simulink model "three_phase_inverter(multi)"  (R2021b)
settings: Solver=FixedStepDiscrete  StartTime=0.0  StopTime=5  FixedStep=1e-6  RelTol=1e-3
libraries: spsIGBTDiodeLib x6, simulink x4, spsVoltageMeasurementLib x4, spsSeriesRLCBranchLib x3, spsCurrentMeasurementLib x1, spsDCVoltageSourceLib x1, spspowerguiLib x1
settings Model: Creator=banof  LastModifiedBy=Devanand Kumar
settings DebuggingCC: UnconnectedInputMsg=none  UnconnectedOutputMsg=none  UnconnectedLineMsg=none
settings ModelReferenceCC: EnableRefExpFcnMdlSchedulingChecks=off
settings RTWCC: DLArmComputeVersion=20.02.1

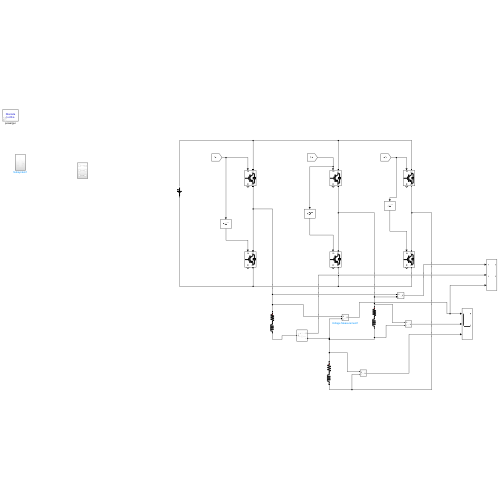
[thumbnail: Simulink's stored preview of the top-level diagram]
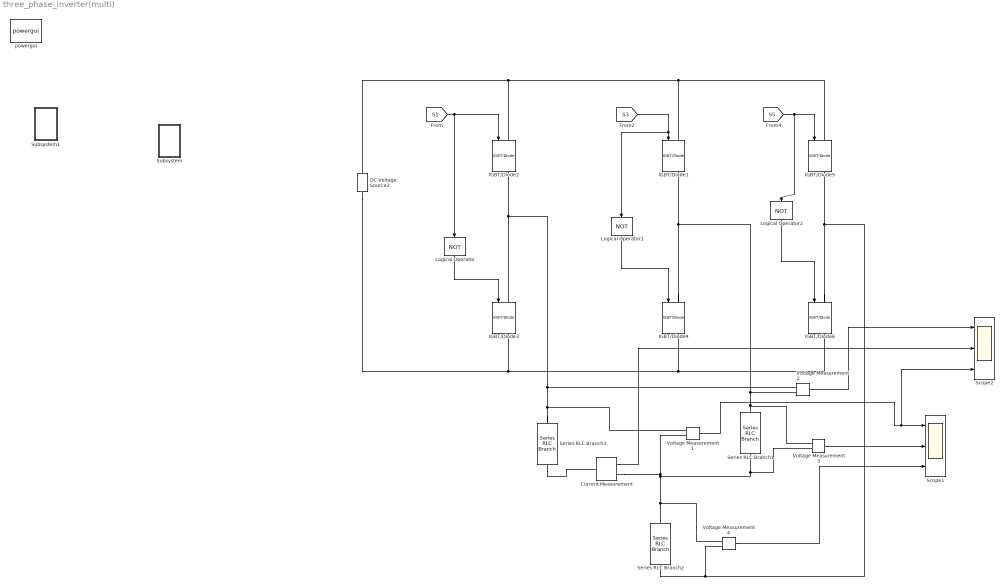
== system three_phase_inverter(multi) ==
  Current Measurement : spsCurrentMeasurementLib/Current Measurement  PhasorSimulation=off  OutputType=Complex  PSBequivalent=0
  DC Voltage Source2 : spsDCVoltageSourceLib/DC Voltage Source  Amplitude=100  Measurements=None
  IGBT/Diode{1..6} (6 alike) : spsIGBTDiodeLib/IGBT//Diode  Ron=1e-3  Rs=1e5  Cs=inf  Measurements=on
  Logical Operator : Logic  Operator=NOT  AllPortsSameDT=off  OutDataTypeStr=boolean
  Logical Operator1 : Logic  Operator=NOT  AllPortsSameDT=off  OutDataTypeStr=boolean
  Logical Operator2 : Logic  Operator=NOT  AllPortsSameDT=off  OutDataTypeStr=boolean
  Scope1 : Scope  NumInputPorts=3
  Scope2 : Scope  NumInputPorts=3
  Series RLC Branch1 : spsSeriesRLCBranchLib/Series RLC Branch  LConnTagsString=__new0  RConnTagsString=__new0  BranchType=RL  Resistance=100  Inductance=100e-3  SetiL0=off  InitialCurrent=0  Capacitance=1e-6  Setx0=off  InitialVoltage=0  Measurements=None
  Series RLC Branch2 : spsSeriesRLCBranchLib/Series RLC Branch  LConnTagsString=__new0  RConnTagsString=__new0  BranchType=RL  Resistance=100  Inductance=100e-3  SetiL0=off  InitialCurrent=0  Capacitance=1e-6  Setx0=off  InitialVoltage=0  Measurements=None
  Series RLC Branch3 : spsSeriesRLCBranchLib/Series RLC Branch  LConnTagsString=__new0  RConnTagsString=__new0  BranchType=RL  Resistance=100  Inductance=100e-3  SetiL0=off  InitialCurrent=0  Capacitance=1e-6  Setx0=off  InitialVoltage=0  Measurements=None
  Subsystem : Subsystem
  Subsystem1 : Subsystem
  Voltage Measurement{1..4} (4 alike) : spsVoltageMeasurementLib/Voltage Measurement  PhasorSimulation=off  OutputType=Complex  PSBequivalent=0
  powergui : spspowerguiLib/powergui  Priority=1  SimulationMode=Discrete  SampleTime=1e-6  frequency=60  Iterations=50  frequencyindice=0  Pbase=100e6  ErrMax=1e-4  UnitsV=kV  UnitsW=MW  buscounter=0  FunctionMessages=off  echomessages=off  EnableUseOfTLC=off  CurrentSourceSwitches=off  DisableSnubberDevices=off  DisableRonSwitches=off  DisableVfSwitches=off  DisplayEquations=off  AutomaticDiscreteSolvers=off  SolverType=Tustin/Backward Euler (TBE)  Interpol=off  ExternalGateDelay=off  methode=off  Ts=100  x0status=blocks  SPID=on  SwTol=0  HookPort=off  NonlinearTolerance=1e-4  nMaxIteration=100  ContinueOnMaxIteration=off  RestoreLinks=warning  ResistiveCurrentMeasurement=off  Frange=[0:2:500]  Ylog=off  Xlog=on  ShowGrid=off  save=off  variable=ZData  structure=0  ZoomFFT=off  StartTime=0.0  cycles=1  DisplayStyle=1  fundamental=60  FreqAxis=off  MaxFrequency=1000  frequencyindicesteady=1  RmsSteady=1  display=off
  wires:
  [S1] -> Logical Operator/1, IGBT/Diode2/1
  Logical Operator/1 -> IGBT/Diode3/1
  [S3] -> Logical Operator1/1, IGBT/Diode1/1
  Logical Operator1/1 -> IGBT/Diode4/1
  Logical Operator2/1 -> IGBT/Diode6/1
  [S5] -> Logical Operator2/1, IGBT/Diode5/1
  Voltage Measurement3/1 -> Scope1/2
  Voltage Measurement1/1 -> Scope2/3, Scope1/1
  Voltage Measurement4/1 -> Scope1/3
  Voltage Measurement2/1 -> Scope2/1
  Current Measurement/1 -> Scope2/2
  connections:
  IGBT/Diode3/RConn1 -- IGBT/Diode6/RConn1 -- IGBT/Diode4/RConn1 -- DC Voltage Source2/LConn1
  IGBT/Diode2/RConn1 -- Voltage Measurement2/LConn1 -- Series RLC Branch3/LConn1 -- Voltage Measurement1/LConn1 -- IGBT/Diode3/LConn1
  DC Voltage Source2/RConn1 -- IGBT/Diode5/LConn1 -- IGBT/Diode1/LConn1 -- IGBT/Diode2/LConn1
  IGBT/Diode4/LConn1 -- Voltage Measurement3/LConn1 -- Series RLC Branch1/LConn1 -- Voltage Measurement2/LConn2 -- IGBT/Diode1/RConn1
  IGBT/Diode6/LConn1 -- Voltage Measurement4/LConn2 -- Series RLC Branch2/RConn1 -- IGBT/Diode5/RConn1
  Voltage Measurement4/LConn1 -- Series RLC Branch2/LConn1 -- Current Measurement/RConn1 -- Voltage Measurement1/LConn2 -- Voltage Measurement3/LConn2 -- Series RLC Branch1/RConn1
  Series RLC Branch3/RConn1 -- Current Measurement/LConn1

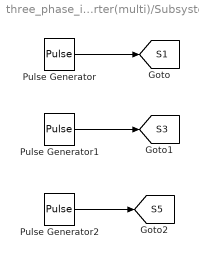
== system three_phase_inverter(multi)/Subsystem ==
  Pulse Generator : DiscretePulseGenerator  Period=20000  PulseWidth=10000  SampleTime=1e-6
  Pulse Generator1 : DiscretePulseGenerator  Period=20000  PulseWidth=10000  PhaseDelay=6666  SampleTime=1e-6
  Pulse Generator2 : DiscretePulseGenerator  Period=20000  PulseWidth=10000  PhaseDelay=13333  SampleTime=1e-6
  tag scope: S1=global, S3=global, S5=global
  wires:
  Pulse Generator/1 -> [S1]
  Pulse Generator2/1 -> [S5]
  Pulse Generator1/1 -> [S3]

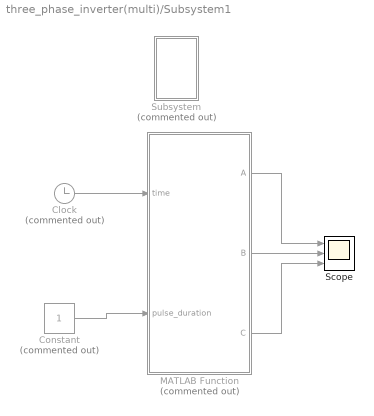
== system three_phase_inverter(multi)/Subsystem1 ==
  Clock : Clock  Commented=on
  Constant : Constant  Commented=on
  MATLAB Function : MATLAB Function  Commented=on  TreatAsAtomicUnit=on
  Scope : Scope  NumInputPorts=3
  Subsystem : Subsystem  Commented=on
  wires:
  MATLAB Function/3(C) -> Scope/3
  Constant/1 -> MATLAB Function/2(pulse_duration)
  MATLAB Function/2(B) -> Scope/2
  MATLAB Function/1(A) -> Scope/1
  Clock/1 -> MATLAB Function/1(time)

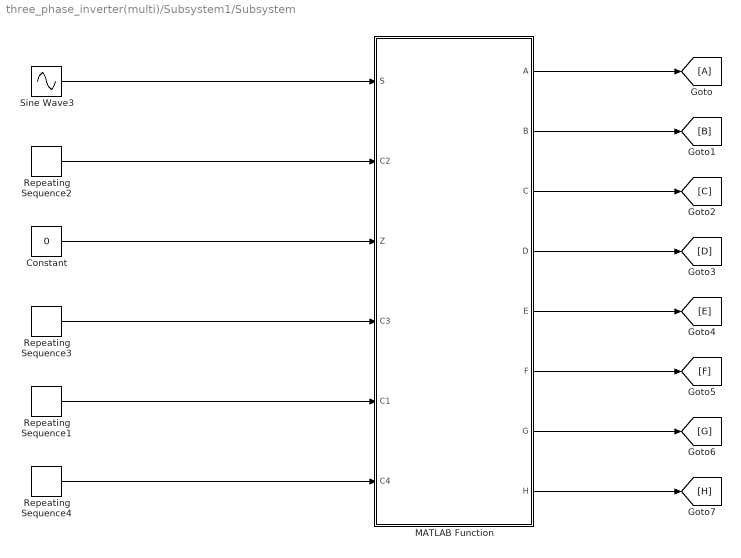
== system three_phase_inverter(multi)/Subsystem1/Subsystem ==
  Constant : Constant  Value=0
  MATLAB Function : MATLAB Function  TreatAsAtomicUnit=on
  Repeating Sequence1 : simulink/Sources/Repeating Sequence  rep_seq_t=[0 0.5/1000 1/1000]  rep_seq_y=[0.5 1 0.5]
  Repeating Sequence2 : simulink/Sources/Repeating Sequence  rep_seq_t=[0 0.5/1000 1/1000]  rep_seq_y=[0 0.5 0]
  Repeating Sequence3 : simulink/Sources/Repeating Sequence  rep_seq_t=[0 0.5/1000 1/1000]  rep_seq_y=[0 -0.5 0]
  Repeating Sequence4 : simulink/Sources/Repeating Sequence  rep_seq_t=[0 0.5/1000 1/1000]  rep_seq_y=[-0.5 -1 -0.5]
  Sine Wave3 : Sin  Frequency=2*pi*50
  wires:
  Repeating Sequence4/1 -> MATLAB Function/6(C4)
  Sine Wave3/1 -> MATLAB Function/1(S)
  Repeating Sequence3/1 -> MATLAB Function/4(C3)
  MATLAB Function/8(H) -> [H]
  MATLAB Function/7(G) -> [G]
  MATLAB Function/5(E) -> [E]
  Repeating Sequence2/1 -> MATLAB Function/2(C2)
  MATLAB Function/1(A) -> [A]
  Constant/1 -> MATLAB Function/3(Z)
  Repeating Sequence1/1 -> MATLAB Function/5(C1)
  MATLAB Function/4(D) -> [D]
  MATLAB Function/2(B) -> [B]
  MATLAB Function/3(C) -> [C]
  MATLAB Function/6(F) -> [F]

== matlab function three_phase_inverter(multi)/Subsystem1/MATLAB Function ==
  data: time input; A output; B output; pulse_duration input; C output
function [A,B,C] = fcn(time, pulse_duration)
    phase_shift = 2*pi/3;
    if mod(time, 1.5*pulse_duration) < pulse_duration
        A = 1;
    else
        A = 0;
    end
    
    if mod(time - phase_shift, 1.5*pulse_duration) < pulse_duration
        B = 1;
    else
        B = 0;
    end
    
    if mod(time - 2*phase_shift, 1.5*pulse_duration) < pulse_duration
        C = 1;
    else
        C = 0;
    end
end

== matlab function three_phase_inverter(multi)/Subsystem1/Subsystem/MATLAB Function ==
  data: S input; C2 input; A output; B output; C output; D output; E output; F output; G output; H output; Z input; C3 input; C1 input; C4 input
function [A,B,C,D,E,F,G,H]= myfcn(S,C2,Z,C3,C1,C4)
    a=0;b=0;c=0;d=0;e=0;f=0;g=0;h=0;
    if S>C2&&S>Z&&S>C1%2Vdc
    a=1;
    b=0;
    c=0;
    d=1;
    e=1;
    f=0;
    g=0;
    h=1;
elseif S<C1&&S>Z&&S>C2%Vdc
    a=1;
    b=0;
    c=0;
    d=1;
    e=1;
    f=0;
    g=1;
    h=0;
    elseif S<C1&&S>Z&&S<C2%0VDC
   a=1;
   b=0;
    c=1;
    d=0;
    e=1;
    f=0;
    g=1;
    h=0;  
  elseif S>C3&&S<Z&&S>C4%0Vdc
    a=1;
    b=0;
    c=1;
    d=0;
    e=1;
    f=0;
    g=1;
    h=0;    
elseif S<C3&&S>C4&&S<Z%-Vdc
    a=0;
    b=1;
    c=1;
    d=0; 
    e=0;
    f=1;
    g=0;
    h=1;
elseif S<C3&&S<Z&&S<C4%-2Vdc
    a=0;
    b=1;
    c=1;
    d=0;
    e=0;
    f=1;
    g=1;
    h=0;
    end
A=a;
B=b;
C=c;
D=d;
E=e;
F=f;
G=g;
H=h;
